simulink model "helicopter_2DOF"  (R2026a)
settings: Solver=VariableStepAuto
values from neighbouring files (symbols this model uses):
  act = getBaseVariable('act')    [run_simulink_simulations.m]
  alpha0 = deg2rad(15)    [1_init.m]    (also in build_uncertain_linear_model.m; init.m; run_simulink_simulations.m = evalin('base','alpha0'))
  Aobs = A - Ke*Cmeas    [2_LQG_2DOF_Synthesis.m]    (also in LQG_2DOF_Synthesis.m; PIDcomp_decoupler_sensitivity.m; run_simulink_simulations.m)
  beta0 = deg2rad(20)    [1_init.m]    (also in build_uncertain_linear_model.m; init.m; run_simulink_simulations.m = evalin('base','beta0'))
  Bobs = [B Ke]    [2_LQG_2DOF_Synthesis.m]    (also in LQG_2DOF_Synthesis.m; PIDcomp_decoupler_sensitivity.m; run_simulink_simulations.m)
  Cobs = eye(size(A))    [2_LQG_2DOF_Synthesis.m]    (also in LQG_2DOF_Synthesis.m; PIDcomp_decoupler_sensitivity.m; run_simulink_simulations.m)
  Ctrack = [ ... (first row only)    [2_LQG_2DOF_Synthesis.m]    (also in LQG_2DOF_Controllers.mat = [0 0 0 0 0 0 0 0 0 0 0 0 ... (20 elements, 2x10)]; LQG_2DOF_Synthesis.m)
  delta_plant = zeros(7,1)    [1_init.m]    (also in 6_HINF_RAS_Simulink.m; init.m)
  Dobs = zeros(size(A,1), size(B,2) + size(Cmeas,1))    [2_LQG_2DOF_Synthesis.m]    (also in LQG_2DOF_Synthesis.m; PIDcomp_decoupler_sensitivity.m = zeros(size(A,1),size(B,2)+size(Cmeas,1)); run_simulink_simulations.m = zeros(size(A,1),size(B,2)+size(Cmeas,1)))
  HINF_controller_id = 1    [1_init.m]    (also in 6_HINF_RAS_Simulink.m = controllerIDs(ic); init.m = 4)
  Hy = (Jsensor.'*Vinv*Jsensor) \      (Jsensor.'*Vinv)    [3_HINF_setup.m]    (also in HINF_setup.m; HINF_setup.mat = [0.105532740103  0  0; 0  -0.00735527189948  -0.020208443457; RAS_vectorized.m = (Jsensor.'*Vinv*Jsensor) \ (Jsensor.'*Vinv))
  K_hinfsyn = minreal(      ss(K_hinfsyn),      1e-7)    [4_HINF_synthesis.m]    (also in HINF_synthesis.m = minreal(          Du *          K_hinfsyn_scaled *          )
  K_LQG = ss(      Ac_LQG,      Bc_LQG,      Cc_LQG,      Dc_LQG)    [2_LQG_2DOF_Synthesis.m]    (also in LQG_2DOF_Synthesis.m)
  K_mix = minreal(      ss(K_mix),      1e-7)    [4_HINF_synthesis.m]    (also in HINF_synthesis.m = minreal(          Du *          K_mix_scaled *          Dy_i)
  Kalpha_tuned = getBlockValue(CLpidTuned,'Kalpha')    [4_HINF_synthesis.m]    (also in HINF_synthesis.m = pid(          alphaScaledToPhys *          Kalpha_tuned_scal)
  Kbeta_tuned = getBlockValue(CLpidTuned,'Kbeta')    [4_HINF_synthesis.m]    (also in HINF_synthesis.m = pid(          betaScaledToPhys *          Kbeta_tuned_scaled)
  Ki_LQGI = Kaug_LQI(:,n+1:end)    [2_LQG_2DOF_Synthesis.m]    (also in LQG_2DOF_Controllers.mat = [-6.12353410994  -0.048270119194; 0.048270119194  -6.1235341; LQG_2DOF_Synthesis.m)
  Kx_LQGI = Kaug_LQI(:,1:n)    [2_LQG_2DOF_Synthesis.m]    (also in LQG_2DOF_Controllers.mat = [2.67945787682 0.0236091239115 4.27147445601 0.0421494721099; LQG_2DOF_Synthesis.m)
  P_nominal = ss(P_uncertain.NominalValue)    [build_uncertain_linear_model.m]
  ref = struct    [run_simulink_simulations.m]
  sensor = getBaseVariable('sensor')    [run_simulink_simulations.m]
  u0 = E0 \ [ ... (first row only)    [1_init.m]    (also in build_uncertain_linear_model.m = u0_nominal; init.m)
  x0 = [alpha0; 0; beta0; 0]    [1_init.m]    (also in build_uncertain_linear_model.m = [; init.m)
  xhat0 = zeros(size(A,1),1)    [2_LQG_2DOF_Synthesis.m]    (also in LQG_2DOF_Synthesis.m; PIDcomp_decoupler_sensitivity.m; run_simulink_simulations.m)
  y0_sensor = [ ... (first row only)    [2_LQG_2DOF_Synthesis.m]    (also in 3_HINF_setup.m; HINF_setup.m; HINF_setup.mat = [2.53901483246 43.6957068665 -15.9039366646]; LQG_2DOF_Controllers.mat = [2.53901483246 43.6957068665 -15.9039366646])
undefined symbols (not defined in the file or in its folder): params
libraries: simulink x4, slpidlib x2, RCTblocks x2
settings Model: Creator=bonci  LastModifiedBy=bonci
settings DebuggingCC: UnderSpecifiedDimensionMsg=warning

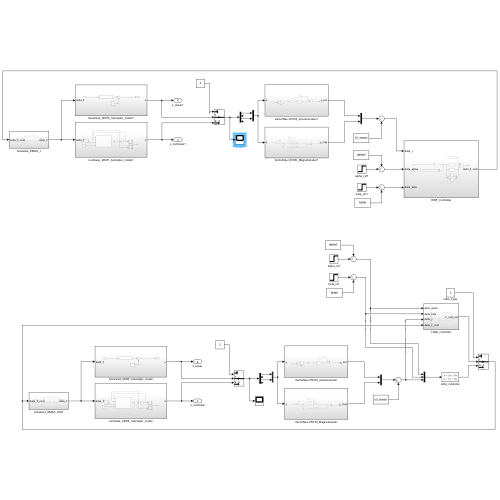
[thumbnail: Simulink's stored preview of the top-level diagram]
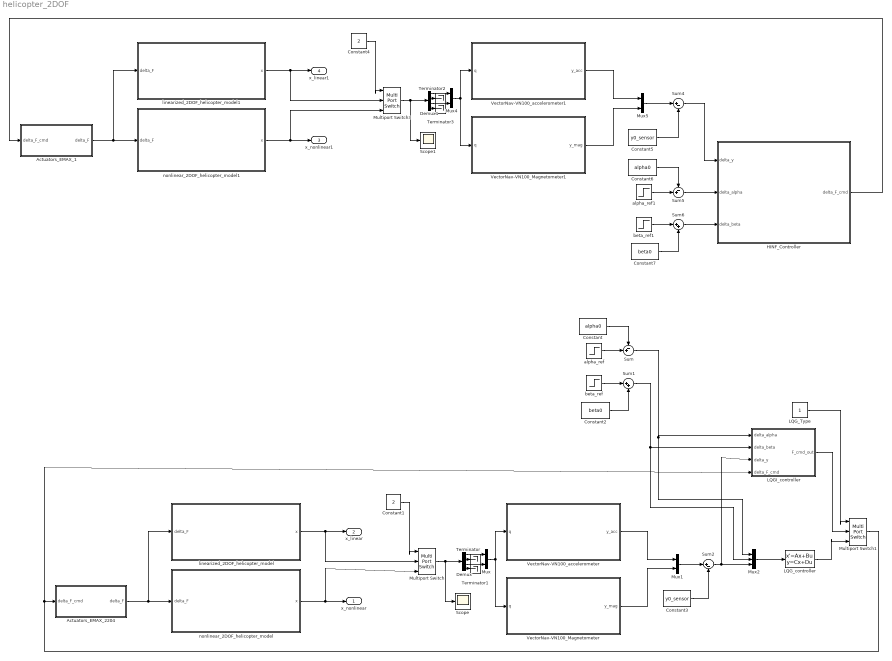
== system helicopter_2DOF ==
  Actuators_EMAX_1 : Subsystem
  Actuators_EMAX_2204 : Subsystem
  Constant : Constant  Value=alpha0
  Constant1 : Constant  Value=2
  Constant2 : Constant  Value=beta0
  Constant3 : Constant  Value=y0_sensor
  Constant4 : Constant  Value=2
  Constant5 : Constant  Value=y0_sensor
  Constant6 : Constant  Value=alpha0
  Constant7 : Constant  Value=beta0
  Demux : Demux
  Demux1 : Demux
  HINF_Controller : Subsystem
  LQGI_controller : Subsystem
  LQG_Type : Constant
  LQG_controller : StateSpace  A=K_LQG.A  B=K_LQG.B  C=K_LQG.C  D=K_LQG.D  InitialCondition=zeros(size(K_LQG.A,1),1)
  Multiport Switch : MultiPortSwitch  Inputs=2  SaturateOnIntegerOverflow=off  InputSameDT=off
  Multiport Switch1 : MultiPortSwitch  Inputs=2  SaturateOnIntegerOverflow=off  InputSameDT=off
  Multiport Switch3 : MultiPortSwitch  Inputs=2  SaturateOnIntegerOverflow=off  InputSameDT=off
  Mux{,1,4..5} (4 alike) : Mux  Inputs=2
  Mux2 : Mux  Inputs=3
  Scope : Scope
      settings: ActiveDisplayYMinimum=0.012690963075634137  ActiveDisplayYMaximum=1.2842322538970823
  Scope1 : Scope
      settings: ActiveDisplayYMinimum=-318.72541889346883  ActiveDisplayYMaximum=39.006233463535438
  Sum : Sum  Inputs=-+|
  Sum1 : Sum  Inputs=|++
  Sum2 : Sum  Inputs=|+-
  Sum4 : Sum  Inputs=|+-
  Sum5 : Sum  Inputs=-+|
  Sum6 : Sum  Inputs=|++
  Terminator{,1..3} (4 alike) : Terminator
  VectorNav-VN100_Magnetometer : Subsystem
  VectorNav-VN100_Magnetometer1 : Subsystem
  VectorNav-VN100_accelerometer : Subsystem
  VectorNav-VN100_accelerometer1 : Subsystem
  alpha_ref : Step  Time=ref.alpha.time  InitialValue=ref.alpha.initial  FinalValue=ref.alpha.final  SampleTime=0
  alpha_ref1 : Step  Time=ref.alpha.time  InitialValue=ref.alpha.initial  FinalValue=ref.alpha.final  SampleTime=0
  beta_ref : Step  Time=ref.beta.time  InitialValue=ref.beta.initial  FinalValue=ref.beta.final  SampleTime=0
  beta_ref1 : Step  Time=ref.beta.time  InitialValue=ref.beta.initial  FinalValue=ref.beta.final  SampleTime=0
  linearized_2DOF_helicopter_model : Subsystem
  linearized_2DOF_helicopter_model1 : Subsystem
  nonlinear_2DOF_helicopter_model : Subsystem
  nonlinear_2DOF_helicopter_model1 : Subsystem
  x_nonlinear : Outport
  x_linear : Outport  Port=2
  x_nonlinear1 : Outport  Port=3
  x_linear1 : Outport  Port=4
  wires:
  nonlinear_2DOF_helicopter_model/1(x) -> Multiport Switch/3, x_nonlinear/1
  linearized_2DOF_helicopter_model/1(x) -> Multiport Switch/2, x_linear/1
  Constant1/1 -> Multiport Switch/1
  Multiport Switch/1 -> Demux/1, Scope/1
  Actuators_EMAX_2204/1(delta_F) -> linearized_2DOF_helicopter_model/1(delta_F), nonlinear_2DOF_helicopter_model/1(delta_F)
  VectorNav-VN100_accelerometer/1(y_acc) -> Mux1/1
  VectorNav-VN100_Magnetometer/1(y_mag) -> Mux1/2
  Demux/1 -> Mux/1
  Demux/3 -> Mux/2
  Mux/1 -> VectorNav-VN100_Magnetometer/1(q), VectorNav-VN100_accelerometer/1(q)
  Demux/2 -> Terminator/1
  Demux/4 -> Terminator1/1
  alpha_ref/1 -> Sum/2
  beta_ref/1 -> Sum1/1
  Constant/1 -> Sum/1
  Constant2/1 -> Sum1/2
  Mux1/1 -> Sum2/1
  Constant3/1 -> Sum2/2
  Sum2/1 -> Mux2/3, LQGI_controller/3(delta_y)
  Sum/1 -> Mux2/1, LQGI_controller/1(delta_alpha)
  Sum1/1 -> LQGI_controller/2(delta_beta), Mux2/2
  Mux2/1 -> LQG_controller/1
  LQG_controller/1 -> Multiport Switch1/3
  LQG_Type/1 -> Multiport Switch1/1
  Multiport Switch1/1 -> Actuators_EMAX_2204/1(delta_F_cmd), LQGI_controller/4(delta_F_cmd)
  LQGI_controller/1(F_cmd_out) -> Multiport Switch1/2
  Mux5/1 -> Sum4/1
  Constant5/1 -> Sum4/2
  VectorNav-VN100_accelerometer1/1(y_acc) -> Mux5/1
  Demux1/1 -> Mux4/1
  VectorNav-VN100_Magnetometer1/1(y_mag) -> Mux5/2
  Mux4/1 -> VectorNav-VN100_Magnetometer1/1(q), VectorNav-VN100_accelerometer1/1(q)
  Demux1/2 -> Terminator2/1
  Actuators_EMAX_1/1(delta_F) -> linearized_2DOF_helicopter_model1/1(delta_F), nonlinear_2DOF_helicopter_model1/1(delta_F)
  Demux1/4 -> Terminator3/1
  Demux1/3 -> Mux4/2
  Constant4/1 -> Multiport Switch3/1
  Multiport Switch3/1 -> Demux1/1, Scope1/1
  linearized_2DOF_helicopter_model1/1(x) -> Multiport Switch3/2, x_linear1/1
  nonlinear_2DOF_helicopter_model1/1(x) -> Multiport Switch3/3, x_nonlinear1/1
  Constant6/1 -> Sum5/1
  alpha_ref1/1 -> Sum5/2
  beta_ref1/1 -> Sum6/1
  Constant7/1 -> Sum6/2
  Sum4/1 -> HINF_Controller/1(delta_y)
  Sum5/1 -> HINF_Controller/2(delta_alpha)
  Sum6/1 -> HINF_Controller/3(delta_beta)
  HINF_Controller/1(delta_F_cmd) -> Actuators_EMAX_1/1(delta_F_cmd)

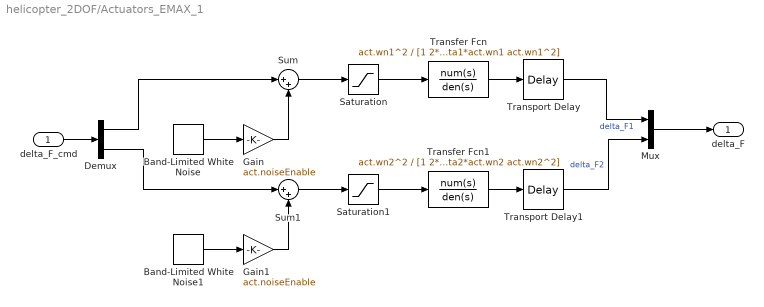
== system helicopter_2DOF/Actuators_EMAX_1 ==
  delta_F_cmd : Inport
  Band-Limited White Noise : simulink/Sources/Band-Limited White Noise  Cov=act.noisePower_F1  Ts=act.Ts_noise  seed=101
  Band-Limited White Noise1 : simulink/Sources/Band-Limited White Noise  Cov=act.noisePower_F2  Ts=act.Ts_noise  seed=202
  Demux : Demux  Outputs=2
  Gain : Gain  Gain=act.noiseEnable
  Gain1 : Gain  Gain=act.noiseEnable
  Mux : Mux  Inputs=2
  Saturation : Saturate  UpperLimit=act.deltaF1_max  LowerLimit=act.deltaF1_min
  Saturation1 : Saturate  UpperLimit=act.deltaF2_max  LowerLimit=act.deltaF2_min
  Sum : Sum  Inputs=|++
  Sum1 : Sum  Inputs=|++
  Transfer Fcn : TransferFcn  Numerator=act.wn1^2  Denominator=[1 2*act.zeta1*act.wn1 act.wn1^2]
  Transfer Fcn1 : TransferFcn  Numerator=act.wn2^2  Denominator=[1 2*act.zeta2*act.wn2 act.wn2^2]
  Transport Delay : TransportDelay  DelayTime=act.td1
  Transport Delay1 : TransportDelay  DelayTime=act.td2
  delta_F : Outport
  wires:
  Gain/1 -> Sum/2
  Saturation1/1 -> Transfer Fcn1/1
  Sum/1 -> Saturation/1
  Mux/1 -> delta_F/1
  Demux/1 -> Sum/1
  Transport Delay/1 -> Mux/1  "delta_F1"
  Transfer Fcn/1 -> Transport Delay/1
  Demux/2 -> Sum1/1
  Transfer Fcn1/1 -> Transport Delay1/1
  Band-Limited White Noise1/1 -> Gain1/1
  Gain1/1 -> Sum1/2
  Sum1/1 -> Saturation1/1
  Transport Delay1/1 -> Mux/2  "delta_F2"
  delta_F_cmd/1 -> Demux/1
  Band-Limited White Noise/1 -> Gain/1
  Saturation/1 -> Transfer Fcn/1

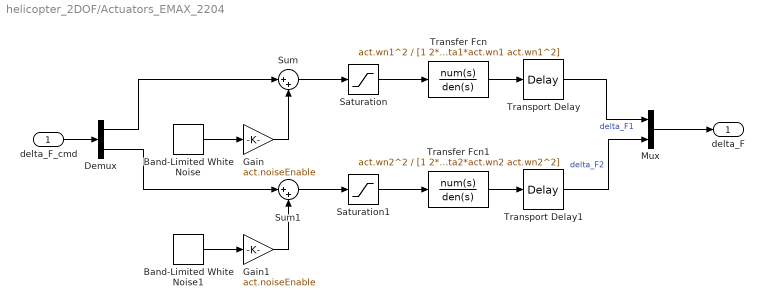
== system helicopter_2DOF/Actuators_EMAX_2204 ==
  delta_F_cmd : Inport
  Band-Limited White Noise : simulink/Sources/Band-Limited White Noise  Cov=act.noisePower_F1  Ts=act.Ts_noise  seed=101
  Band-Limited White Noise1 : simulink/Sources/Band-Limited White Noise  Cov=act.noisePower_F2  Ts=act.Ts_noise  seed=202
  Demux : Demux  Outputs=2
  Gain : Gain  Gain=act.noiseEnable
  Gain1 : Gain  Gain=act.noiseEnable
  Mux : Mux  Inputs=2
  Saturation : Saturate  UpperLimit=act.deltaF1_max  LowerLimit=act.deltaF1_min
  Saturation1 : Saturate  UpperLimit=act.deltaF2_max  LowerLimit=act.deltaF2_min
  Sum : Sum  Inputs=|++
  Sum1 : Sum  Inputs=|++
  Transfer Fcn : TransferFcn  Numerator=act.wn1^2  Denominator=[1 2*act.zeta1*act.wn1 act.wn1^2]
  Transfer Fcn1 : TransferFcn  Numerator=act.wn2^2  Denominator=[1 2*act.zeta2*act.wn2 act.wn2^2]
  Transport Delay : TransportDelay  DelayTime=act.td1
  Transport Delay1 : TransportDelay  DelayTime=act.td2
  delta_F : Outport
  wires:
  Gain/1 -> Sum/2
  Saturation1/1 -> Transfer Fcn1/1
  Sum/1 -> Saturation/1
  Mux/1 -> delta_F/1
  Demux/1 -> Sum/1
  Transport Delay/1 -> Mux/1  "delta_F1"
  Transfer Fcn/1 -> Transport Delay/1
  Demux/2 -> Sum1/1
  Transfer Fcn1/1 -> Transport Delay1/1
  Band-Limited White Noise1/1 -> Gain1/1
  Gain1/1 -> Sum1/2
  Sum1/1 -> Saturation1/1
  Transport Delay1/1 -> Mux/2  "delta_F2"
  delta_F_cmd/1 -> Demux/1
  Band-Limited White Noise/1 -> Gain/1
  Saturation/1 -> Transfer Fcn/1

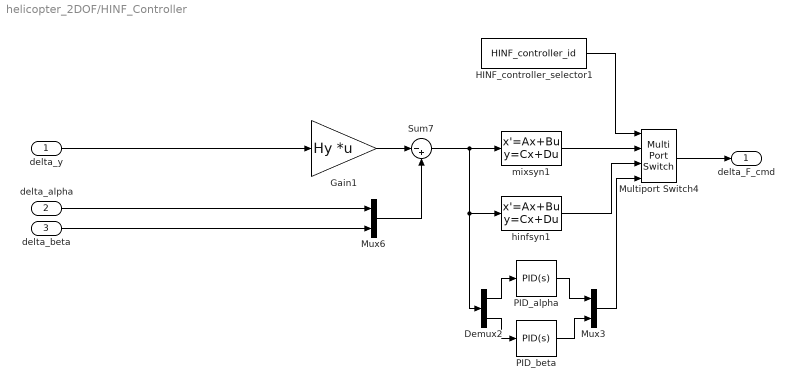
== system helicopter_2DOF/HINF_Controller ==
  delta_y : Inport
  delta_alpha : Inport  Port=2
  delta_beta : Inport  Port=3
  Demux2 : Demux  Outputs=2
  Gain1 : Gain  Gain=Hy  Multiplication=Matrix(K*u)
  HINF_controller_selector1 : Constant  Value=HINF_controller_id
  Multiport Switch4 : MultiPortSwitch  SaturateOnIntegerOverflow=off  InputSameDT=off
  Mux3 : Mux  Inputs=2
  Mux6 : Mux  Inputs=2
  PID_alpha : slpidlib/PID Controller  Controller=PID  Form=Parallel  TimeDomain=Continuous-time  UseExternalTs=off  SampleTime=-1  IntegratorMethod=Forward Euler  FilterMethod=Forward Euler  ControllerParametersSource=internal  P=Kalpha_tuned.Kp  I=Kalpha_tuned.Ki  UseKiTs=off  D=Kalpha_tuned.Kd  UseExternalDerivativeSource=off  N=1/Kalpha_tuned.Tf  UseFilter=on  TunerSelectOption=Transfer Function Based (PID Tuner App)  InitialConditionSource=internal  InitialConditionForIntegrator=0  InitialConditionForFilter=0  DifferentiatorICPrevScaledInput=0  ExternalReset=none  TrackingMode=off  Kt=1  LimitOutput=off  SatLimitsSource=internal  UpperSaturationLimit=inf  LowerSaturationLimit=-inf  LinearizeAsGain=on  AntiWindupMode=none  Kb=1  LimitIntegrator=off  UpperIntegratorSaturationLimit=inf  LowerIntegratorSaturationLimit=-inf  POutMin=[]  POutMax=[]  IOutMin=[]  IOutMax=[]  DOutMin=[]  DOutMax=[]  NOutMin=[]  NOutMax=[]  SumOutMin=[]  SumOutMax=[]  SaturationOutMin=[]  SaturationOutMax=[]  PParamMin=[]  PParamMax=[]  IParamMin=[]  IParamMax=[]  DParamMin=[]  DParamMax=[]  NParamMin=[]  NParamMax=[]  KbParamMin=[]  KbParamMax=[]  KtParamMin=[]  KtParamMax=[]  KbOutMin=[]  KbOutMax=[]  KtOutMin=[]  KtOutMax=[]  IntegratorOutMin=[]  IntegratorOutMax=[]  FilterOutMin=[]  FilterOutMax=[]  SumI1OutMin=[]  SumI1OutMax=[]  SumI2OutMin=[]  SumI2OutMax=[]  SumI3OutMin=[]  SumI3OutMax=[]  SumI4OutMin=[]  SumI4OutMax=[]  SumDOutMin=[]  SumDOutMax=[]  DifferentiatorOutMin=[]  DifferentiatorOutMax=[]  FilterDiffOutCoefMin=[]  FilterDiffOutCoefMax=[]  ReciprocalOutMin=[]  ReciprocalOutMax=[]  SumDenOutMin=[]  SumDenOutMax=[]  SumNumOutMin=[]  SumNumOutMax=[]  DivideOutMin=[]  DivideOutMax=[]  UdiffTsProdOutMin=[]  UdiffTsProdOutMax=[]  NTsProdOutMin=[]  NTsProdOutMax=[]  UintegralTsProdOutMin=[]  UintegralTsProdOutMax=[]  UngainTsProdOutMin=[]  UngainTsProdOutMax=[]  ClampingZeroOutDataTypeStr=Inherit: Inherit via back propagation  ClampingZeroOutMin=[]  ClampingZeroOutMax=[]  FilterDenConstantOutDataTypeStr=Inherit: Inherit via back propagation  FilterDenConstantOutMin=[]  FilterDenConstantOutMax=[]  PCopyOutDataTypeStr=Inherit: Inherit via back propagation  PCopyOutMin=[]  PCopyOutMax=[]  NCopyOutDataTypeStr=Inherit: Inherit via back propagation  NCopyOutMin=[]  NCopyOutMax=[]  IntegratorContinuousStateAttributes=''  IntegratorStateMustResolveToSignalObject=off  IntegratorRTWStateStorageClass=Auto  FilterContinuousStateAttributes=''  FilterStateMustResolveToSignalObject=off  FilterRTWStateStorageClass=Auto  ParallelPVariant=InternalParameters  IdealPVariant=Disabled  IVariant=InternalParameters  DVariant=InternalParameters  IntegratorVariant=Continuous  SatVariant=Disabled  AWVariant=Passthrough  PCopyVariant=Disabled  TRVariant=Disabled  FdbkBlocksVariant=Forward  IdealPFdbkVariant=Disabled  SatFdbkVariant=Disabled  DerivativeFilterVariant=ContFilter  NVariant=InternalParameters  NCopyVariant=Disabled  FilterICVariant=InternalICsFilter  IntegratorICVariant=InternalICs  ExternalResetVariant=Disabled  TRSumVariant=Passthrough  SumFdbkVariant=Disabled  SumVariant=Sum_PID  TsampFilterVariant=InternalTs  TsampNgainVariant=Passthrough  TsampIntegralVariant=Disabled_SignalSpec  ExternalSaturationOutDataTypeStr=Inherit: Same as second input  DerivativeSourceVariant=ErrorSignal  PreIntVariant=InternalPreInt
  PID_beta : slpidlib/PID Controller  Controller=PID  Form=Parallel  TimeDomain=Continuous-time  UseExternalTs=off  SampleTime=-1  IntegratorMethod=Forward Euler  FilterMethod=Forward Euler  ControllerParametersSource=internal  P=Kbeta_tuned.Kp  I=Kbeta_tuned.Ki  UseKiTs=off  D=Kbeta_tuned.Kd  UseExternalDerivativeSource=off  N=1/Kbeta_tuned.Tf  UseFilter=on  TunerSelectOption=Transfer Function Based (PID Tuner App)  InitialConditionSource=internal  InitialConditionForIntegrator=0  InitialConditionForFilter=0  DifferentiatorICPrevScaledInput=0  ExternalReset=none  TrackingMode=off  Kt=1  LimitOutput=off  SatLimitsSource=internal  UpperSaturationLimit=inf  LowerSaturationLimit=-inf  LinearizeAsGain=on  AntiWindupMode=none  Kb=1  LimitIntegrator=off  UpperIntegratorSaturationLimit=inf  LowerIntegratorSaturationLimit=-inf  POutMin=[]  POutMax=[]  IOutMin=[]  IOutMax=[]  DOutMin=[]  DOutMax=[]  NOutMin=[]  NOutMax=[]  SumOutMin=[]  SumOutMax=[]  SaturationOutMin=[]  SaturationOutMax=[]  PParamMin=[]  PParamMax=[]  IParamMin=[]  IParamMax=[]  DParamMin=[]  DParamMax=[]  NParamMin=[]  NParamMax=[]  KbParamMin=[]  KbParamMax=[]  KtParamMin=[]  KtParamMax=[]  KbOutMin=[]  KbOutMax=[]  KtOutMin=[]  KtOutMax=[]  IntegratorOutMin=[]  IntegratorOutMax=[]  FilterOutMin=[]  FilterOutMax=[]  SumI1OutMin=[]  SumI1OutMax=[]  SumI2OutMin=[]  SumI2OutMax=[]  SumI3OutMin=[]  SumI3OutMax=[]  SumI4OutMin=[]  SumI4OutMax=[]  SumDOutMin=[]  SumDOutMax=[]  DifferentiatorOutMin=[]  DifferentiatorOutMax=[]  FilterDiffOutCoefMin=[]  FilterDiffOutCoefMax=[]  ReciprocalOutMin=[]  ReciprocalOutMax=[]  SumDenOutMin=[]  SumDenOutMax=[]  SumNumOutMin=[]  SumNumOutMax=[]  DivideOutMin=[]  DivideOutMax=[]  UdiffTsProdOutMin=[]  UdiffTsProdOutMax=[]  NTsProdOutMin=[]  NTsProdOutMax=[]  UintegralTsProdOutMin=[]  UintegralTsProdOutMax=[]  UngainTsProdOutMin=[]  UngainTsProdOutMax=[]  ClampingZeroOutDataTypeStr=Inherit: Inherit via back propagation  ClampingZeroOutMin=[]  ClampingZeroOutMax=[]  FilterDenConstantOutDataTypeStr=Inherit: Inherit via back propagation  FilterDenConstantOutMin=[]  FilterDenConstantOutMax=[]  PCopyOutDataTypeStr=Inherit: Inherit via back propagation  PCopyOutMin=[]  PCopyOutMax=[]  NCopyOutDataTypeStr=Inherit: Inherit via back propagation  NCopyOutMin=[]  NCopyOutMax=[]  IntegratorContinuousStateAttributes=''  IntegratorStateMustResolveToSignalObject=off  IntegratorRTWStateStorageClass=Auto  FilterContinuousStateAttributes=''  FilterStateMustResolveToSignalObject=off  FilterRTWStateStorageClass=Auto  ParallelPVariant=InternalParameters  IdealPVariant=Disabled  IVariant=InternalParameters  DVariant=InternalParameters  IntegratorVariant=Continuous  SatVariant=Disabled  AWVariant=Passthrough  PCopyVariant=Disabled  TRVariant=Disabled  FdbkBlocksVariant=Forward  IdealPFdbkVariant=Disabled  SatFdbkVariant=Disabled  DerivativeFilterVariant=ContFilter  NVariant=InternalParameters  NCopyVariant=Disabled  FilterICVariant=InternalICsFilter  IntegratorICVariant=InternalICs  ExternalResetVariant=Disabled  TRSumVariant=Passthrough  SumFdbkVariant=Disabled  SumVariant=Sum_PID  TsampFilterVariant=InternalTs  TsampNgainVariant=Passthrough  TsampIntegralVariant=Disabled_SignalSpec  ExternalSaturationOutDataTypeStr=Inherit: Same as second input  DerivativeSourceVariant=ErrorSignal  PreIntVariant=InternalPreInt
  Sum7 : Sum  Inputs=|-+
  hinfsyn1 : StateSpace  A=K_hinfsyn.A  B=K_hinfsyn.B  C=K_hinfsyn.C  D=K_hinfsyn.D  InitialCondition=zeros(size(K_hinfsyn.A,1),1)
  mixsyn1 : StateSpace  A=K_mix.A  B=K_mix.B  C=K_mix.C  D=K_mix.D  InitialCondition=zeros(size(K_mix.A,1),1)
  delta_F_cmd : Outport
  wires:
  Gain1/1 -> Sum7/1
  Sum7/1 -> hinfsyn1/1, Demux2/1, mixsyn1/1
  Mux6/1 -> Sum7/2
  Mux3/1 -> Multiport Switch4/4
  mixsyn1/1 -> Multiport Switch4/2
  HINF_controller_selector1/1 -> Multiport Switch4/1
  PID_alpha/1 -> Mux3/1
  hinfsyn1/1 -> Multiport Switch4/3
  delta_y/1 -> Gain1/1
  Demux2/1 -> PID_alpha/1
  PID_beta/1 -> Mux3/2
  Demux2/2 -> PID_beta/1
  delta_alpha/1 -> Mux6/1
  Multiport Switch4/1 -> delta_F_cmd/1
  delta_beta/1 -> Mux6/2

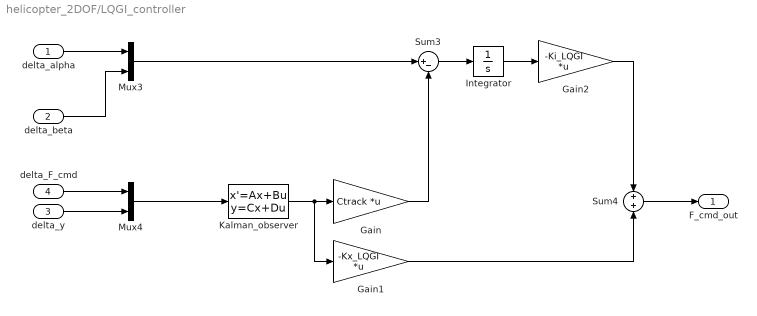
== system helicopter_2DOF/LQGI_controller ==
  delta_alpha : Inport
  delta_beta : Inport  Port=2
  delta_y : Inport  Port=3
  delta_F_cmd : Inport  Port=4
  Gain : Gain  Gain=Ctrack  Multiplication=Matrix(K*u)
  Gain1 : Gain  Gain=-Kx_LQGI  Multiplication=Matrix(K*u)
  Gain2 : Gain  Gain=-Ki_LQGI  Multiplication=Matrix(K*u)
  Integrator : Integrator  InitialCondition=zeros(2,1)
  Kalman_observer : StateSpace  A=Aobs  B=Bobs  C=Cobs  D=Dobs  InitialCondition=xhat0
  Mux3 : Mux  Inputs=2
  Mux4 : Mux  Inputs=2
  Sum3 : Sum  Inputs=|+-
  Sum4 : Sum  Inputs=+|+
  F_cmd_out : Outport
  wires:
  Gain2/1 -> Sum4/1
  Mux3/1 -> Sum3/1
  Sum3/1 -> Integrator/1
  Gain1/1 -> Sum4/2
  Kalman_observer/1 -> Gain1/1, Gain/1
  delta_F_cmd/1 -> Mux4/1
  delta_y/1 -> Mux4/2
  Gain/1 -> Sum3/2
  Integrator/1 -> Gain2/1
  Mux4/1 -> Kalman_observer/1
  Sum4/1 -> F_cmd_out/1
  delta_alpha/1 -> Mux3/1
  delta_beta/1 -> Mux3/2

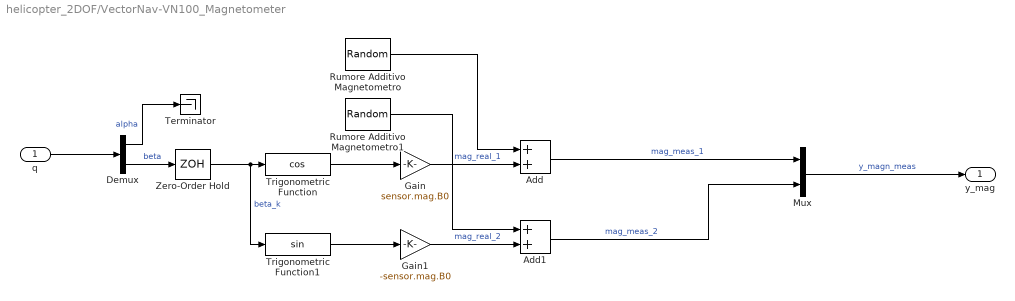
== system helicopter_2DOF/VectorNav-VN100_Magnetometer ==
  q : Inport
  Add : Sum
  Add1 : Sum
  Demux : Demux  Outputs=2
  Gain : Gain  Gain=sensor.mag.B0
  Gain1 : Gain  Gain=-sensor.mag.B0
  Mux : Mux  Inputs=2
  Rumore Additivo Magnetometro : RandomNumber  Variance=sensor.mag.var  Seed=sensor.seed + 1  SampleTime=sensor.mag.Ts
  Rumore Additivo Magnetometro1 : RandomNumber  Variance=sensor.mag.var  Seed=sensor.seed + 300  SampleTime=sensor.mag.Ts
  Terminator : Terminator
  Trigonometric Function : Trigonometry  Operator=cos
  Trigonometric Function1 : Trigonometry
  Zero-Order Hold : ZeroOrderHold  SampleTime=sensor.mag.Ts
  y_mag : Outport
  wires:
  q/1 -> Demux/1
  Demux/2 -> Zero-Order Hold/1  "beta"
  Demux/1 -> Terminator/1  "alpha"
  Trigonometric Function/1 -> Gain/1
  Trigonometric Function1/1 -> Gain1/1
  Gain/1 -> Add/2  "mag_real_1"
  Rumore Additivo Magnetometro/1 -> Add/1
  Gain1/1 -> Add1/2  "mag_real_2"
  Zero-Order Hold/1 -> Trigonometric Function1/1, Trigonometric Function/1  "beta_k"
  Mux/1 -> y_mag/1  "y_magn_meas"
  Add/1 -> Mux/1  "mag_meas_1"
  Rumore Additivo Magnetometro1/1 -> Add1/1
  Add1/1 -> Mux/2  "mag_meas_2"

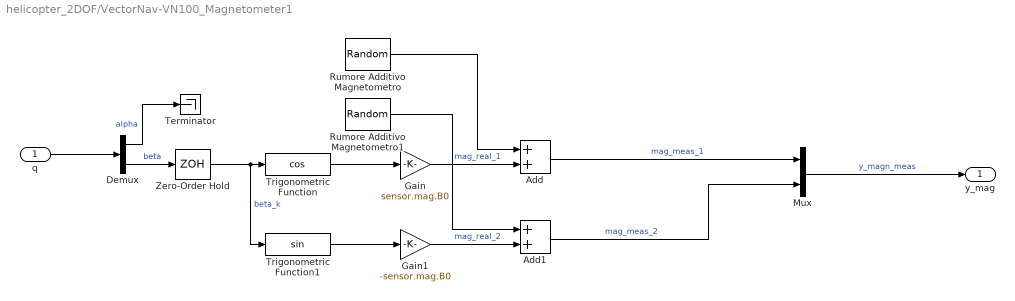
== system helicopter_2DOF/VectorNav-VN100_Magnetometer1 ==
  q : Inport
  Add : Sum
  Add1 : Sum
  Demux : Demux  Outputs=2
  Gain : Gain  Gain=sensor.mag.B0
  Gain1 : Gain  Gain=-sensor.mag.B0
  Mux : Mux  Inputs=2
  Rumore Additivo Magnetometro : RandomNumber  Variance=sensor.mag.var  Seed=sensor.seed + 1  SampleTime=sensor.mag.Ts
  Rumore Additivo Magnetometro1 : RandomNumber  Variance=sensor.mag.var  Seed=sensor.seed + 300  SampleTime=sensor.mag.Ts
  Terminator : Terminator
  Trigonometric Function : Trigonometry  Operator=cos
  Trigonometric Function1 : Trigonometry
  Zero-Order Hold : ZeroOrderHold  SampleTime=sensor.mag.Ts
  y_mag : Outport
  wires:
  q/1 -> Demux/1
  Demux/2 -> Zero-Order Hold/1  "beta"
  Demux/1 -> Terminator/1  "alpha"
  Trigonometric Function/1 -> Gain/1
  Trigonometric Function1/1 -> Gain1/1
  Gain/1 -> Add/2  "mag_real_1"
  Rumore Additivo Magnetometro/1 -> Add/1
  Gain1/1 -> Add1/2  "mag_real_2"
  Zero-Order Hold/1 -> Trigonometric Function1/1, Trigonometric Function/1  "beta_k"
  Mux/1 -> y_mag/1  "y_magn_meas"
  Add/1 -> Mux/1  "mag_meas_1"
  Rumore Additivo Magnetometro1/1 -> Add1/1
  Add1/1 -> Mux/2  "mag_meas_2"

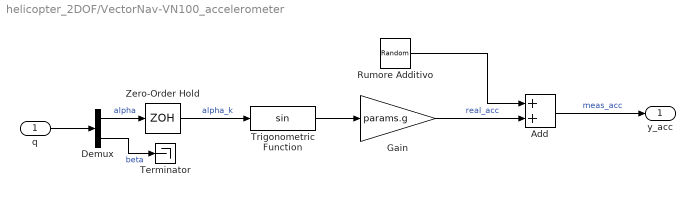
== system helicopter_2DOF/VectorNav-VN100_accelerometer ==
  q : Inport
  Add : Sum
  Demux : Demux  Outputs=2
  Gain : Gain  Gain=params.g
  Rumore Additivo : RandomNumber  Variance=sensor.acc.var  Seed=sensor.seed  SampleTime=sensor.acc.Ts
  Terminator : Terminator
  Trigonometric Function : Trigonometry
  Zero-Order Hold : ZeroOrderHold  SampleTime=sensor.acc.Ts
  y_acc : Outport
  wires:
  q/1 -> Demux/1
  Demux/1 -> Zero-Order Hold/1  "alpha"
  Demux/2 -> Terminator/1  "beta"
  Trigonometric Function/1 -> Gain/1
  Gain/1 -> Add/2  "real_acc"
  Rumore Additivo/1 -> Add/1
  Add/1 -> y_acc/1  "meas_acc"
  Zero-Order Hold/1 -> Trigonometric Function/1  "alpha_k"

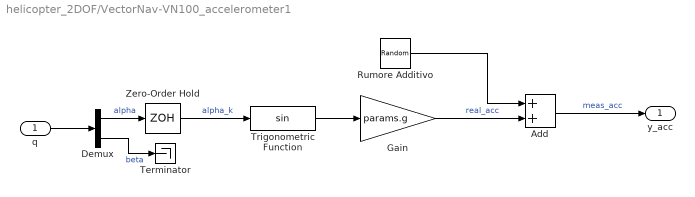
== system helicopter_2DOF/VectorNav-VN100_accelerometer1 ==
  q : Inport
  Add : Sum
  Demux : Demux  Outputs=2
  Gain : Gain  Gain=params.g
  Rumore Additivo : RandomNumber  Variance=sensor.acc.var  Seed=sensor.seed  SampleTime=sensor.acc.Ts
  Terminator : Terminator
  Trigonometric Function : Trigonometry
  Zero-Order Hold : ZeroOrderHold  SampleTime=sensor.acc.Ts
  y_acc : Outport
  wires:
  q/1 -> Demux/1
  Demux/1 -> Zero-Order Hold/1  "alpha"
  Demux/2 -> Terminator/1  "beta"
  Trigonometric Function/1 -> Gain/1
  Gain/1 -> Add/2  "real_acc"
  Rumore Additivo/1 -> Add/1
  Add/1 -> y_acc/1  "meas_acc"
  Zero-Order Hold/1 -> Trigonometric Function/1  "alpha_k"

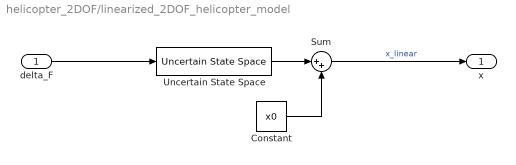
== system helicopter_2DOF/linearized_2DOF_helicopter_model ==
  delta_F : Inport
  Constant : Constant  Value=x0
  Sum : Sum  Inputs=|++
  Uncertain State Space : RCTblocks/Uncertain State Space  Tag=USS  USystem=ss(P_nominal.A,P_nominal.B,eye(4),zeros(4,2))  UValue=[]  X0=zeros(4,1)  uX0=[]
  x : Outport
  wires:
  Uncertain State Space/1 -> Sum/1
  delta_F/1 -> Uncertain State Space/1
  Constant/1 -> Sum/2
  Sum/1 -> x/1  "x_linear"

== system helicopter_2DOF/linearized_2DOF_helicopter_model1 ==
  delta_F : Inport
  Constant : Constant  Value=x0
  Sum : Sum  Inputs=|++
  Uncertain State Space : RCTblocks/Uncertain State Space  Tag=USS  USystem=ss(P_nominal.A,P_nominal.B,eye(4),zeros(4,2))  UValue=[]  X0=zeros(4,1)  uX0=[]
  x : Outport
  wires:
  Uncertain State Space/1 -> Sum/1
  delta_F/1 -> Uncertain State Space/1
  Constant/1 -> Sum/2
  Sum/1 -> x/1  "x_linear"

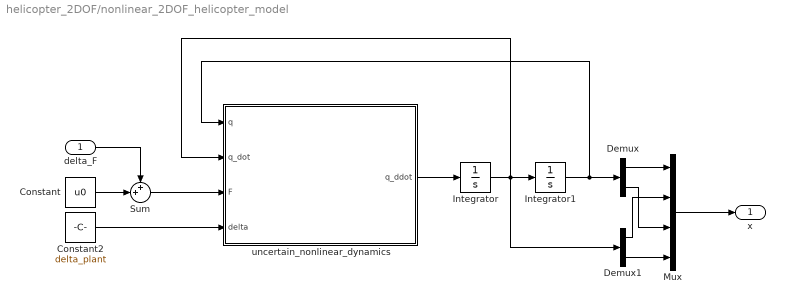
== system helicopter_2DOF/nonlinear_2DOF_helicopter_model ==
  delta_F : Inport
  Constant : Constant  Value=u0
  Constant2 : Constant  Value=delta_plant
  Demux : Demux  Outputs=2
  Demux1 : Demux  Outputs=2
  Integrator : Integrator  InitialCondition=[0 ; 0]
  Integrator1 : Integrator  InitialCondition=[alpha0;beta0]
  Mux : Mux
  Sum : Sum  Inputs=++|
  uncertain_nonlinear_dynamics : MATLAB Function  TreatAsAtomicUnit=on
  x : Outport
  wires:
  Demux1/1 -> Mux/2
  Sum/1 -> uncertain_nonlinear_dynamics/3(F)
  Constant2/1 -> uncertain_nonlinear_dynamics/4(delta)
  Mux/1 -> x/1
  Demux/1 -> Mux/1
  Integrator1/1 -> uncertain_nonlinear_dynamics/1(q), Demux/1
  Demux1/2 -> Mux/4
  uncertain_nonlinear_dynamics/1(q_ddot) -> Integrator/1
  Integrator/1 -> uncertain_nonlinear_dynamics/2(q_dot), Integrator1/1, Demux1/1
  Demux/2 -> Mux/3
  delta_F/1 -> Sum/1
  Constant/1 -> Sum/2

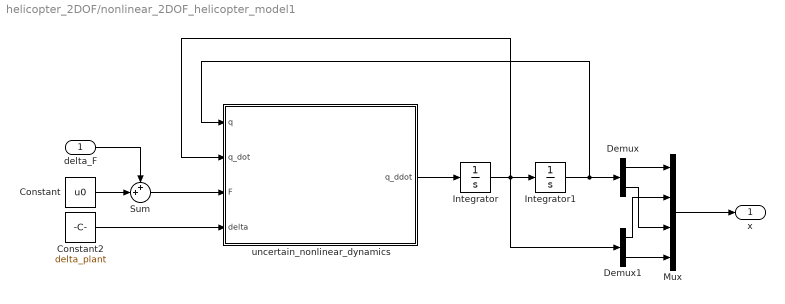
== system helicopter_2DOF/nonlinear_2DOF_helicopter_model1 ==
  delta_F : Inport
  Constant : Constant  Value=u0
  Constant2 : Constant  Value=delta_plant
  Demux : Demux  Outputs=2
  Demux1 : Demux  Outputs=2
  Integrator : Integrator  InitialCondition=[0 ; 0]
  Integrator1 : Integrator  InitialCondition=[alpha0;beta0]
  Mux : Mux
  Sum : Sum  Inputs=++|
  uncertain_nonlinear_dynamics : MATLAB Function  TreatAsAtomicUnit=on
  x : Outport
  wires:
  Demux1/1 -> Mux/2
  Sum/1 -> uncertain_nonlinear_dynamics/3(F)
  Constant2/1 -> uncertain_nonlinear_dynamics/4(delta)
  Mux/1 -> x/1
  Demux/1 -> Mux/1
  Integrator1/1 -> uncertain_nonlinear_dynamics/1(q), Demux/1
  Demux1/2 -> Mux/4
  uncertain_nonlinear_dynamics/1(q_ddot) -> Integrator/1
  Integrator/1 -> uncertain_nonlinear_dynamics/2(q_dot), Integrator1/1, Demux1/1
  Demux/2 -> Mux/3
  delta_F/1 -> Sum/1
  Constant/1 -> Sum/2

== matlab function helicopter_2DOF/nonlinear_2DOF_helicopter_model1/uncertain_nonlinear_dynamics ==
  data: q input; q_ddot output; q_dot input; F input; delta input
function q_ddot = nonlinear_uncertain_dynamics(q, q_dot, F, delta)

    p0.J_alpha = 0.012;       % kg m^2
    p0.J_y = 0.00023;         % kg m^2
    p0.J_z = 0.00364;         % kg m^2
    p0.I_b = 0.00023;         % kg m^2
    
    p0.m = 0.2;               % kg
    p0.l = 0.2;               % m
    
    p0.c_alpha = 0.01;        % N m s/rad
    p0.c_beta  = 0.01;        % N m s/rad
    
    p0.epsilon_p = 0.1;
    p0.epsilon_y = 0.1;
    
    p0.g = 9.81;              % m/s^2
    q_ddot = fcn(q, q_dot, F, delta, p0);
end

== matlab function helicopter_2DOF/nonlinear_2DOF_helicopter_model/uncertain_nonlinear_dynamics ==
  data: q input; q_ddot output; q_dot input; F input; delta input
function q_ddot = nonlinear_uncertain_dynamics(q, q_dot, F, delta)

    p0.J_alpha = 0.012;       % kg m^2
    p0.J_y = 0.00023;         % kg m^2
    p0.J_z = 0.00364;         % kg m^2
    p0.I_b = 0.00023;         % kg m^2
    
    p0.m = 0.2;               % kg
    p0.l = 0.2;               % m
    
    p0.c_alpha = 0.01;        % N m s/rad
    p0.c_beta  = 0.01;        % N m s/rad
    
    p0.epsilon_p = 0.1;
    p0.epsilon_y = 0.1;
    
    p0.g = 9.81;              % m/s^2
    q_ddot = fcn(q, q_dot, F, delta, p0);
end
